simulink model "CRC_8"  (R2018a)
settings: Solver=VariableStepAuto  StartTime=0.0  StopTime=10.0  RelTol=1e-3
values from neighbouring files (symbols this model uses):
  BER = ber(ii)    [CRC_88.m]    (also in RS_77.m)
undefined symbols (not defined in the file or in its folder): CRC
libraries: commcrc2 x2, commrandsrc3 x1, commchan3 x1, dspmathops x1, commsink2 x1
settings Model: Creator=sdf  LastModifiedBy=sdf

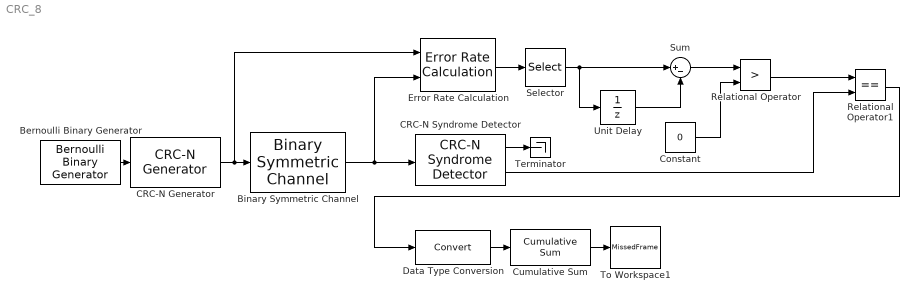
== system CRC_8 ==
  Bernoulli Binary Generator : commrandsrc3/Bernoulli Binary Generator  ProbabilityOfZero=0.5  SeedSource=Parameter  Seed=61  SampleTime=1/640000  SamplesPerFrame=64  OutputDataType=double  SimulateUsing=Interpreted execution
  Binary Symmetric Channel : commchan3/Binary Symmetric Channel  P=BER  s=71  E=off  outDtype=double
      settings: SourceProductName=Communications System Toolbox  SourceProductBaseCode=CM
  CRC-N Generator : commcrc2/CRC-N Generator  crcMethod=CRC-16  iniStates=[0]  numChecksums=1
      settings: SourceProductName=Communications System Toolbox  SourceProductBaseCode=CM
  CRC-N Syndrome Detector : commcrc2/CRC-N Syndrome Detector  crcMethod=CRC-16  iniStates=[0]  numChecksums=1
      settings: SourceProductName=Communications System Toolbox  SourceProductBaseCode=CM
  Constant : Constant  Value=0
  Cumulative Sum : dspmathops/Cumulative Sum  dim=Channels (running sum)  InputProcessing=Columns as channels (frame based)  reset_popup=None  roundingMode=Floor  overflowMode=off  outputDataTypeStr=Inherit: Same as accumulator  outputMin=[]  outputMax=[]  outputLastDataTypeStr=Inherit: Same as accumulator
      settings: SourceProductName=DSP System Toolbox
  Data Type Conversion : DataTypeConversion
  Error Rate Calculation : commsink2/Error Rate Calculation  N=0  st_delay=0  cp_mode=Entire frame  subframe=[]  PMode=Port  WsName=ErrorVec  RsMode2=off  stop=off  numErr=100  maxBits=1e6
  Relational Operator : RelationalOperator  Operator=>  OutDataTypeStr=boolean  RndMeth=Simplest
  Relational Operator1 : RelationalOperator  Operator===  OutDataTypeStr=boolean  RndMeth=Simplest
  Selector : Selector  InputPortWidth=3  IndexOptions=Index vector (dialog)  Indices=[1 3]  OutputSizes=1
  Sum : Sum  Inputs=|+-
  Terminator : Terminator
  To Workspace1 : ToWorkspace  VariableName=MissedFrame  SampleTime=-1
      settings: Save2DSignal=2-D array (concatenate along first dimension)
  Unit Delay : UnitDelay  SampleTime=-1
  wires:
  CRC-N Generator/1 -> Error Rate Calculation/1, Binary Symmetric Channel/1
  Bernoulli Binary Generator/1 -> CRC-N Generator/1
  Binary Symmetric Channel/1 -> Error Rate Calculation/2, CRC-N Syndrome Detector/1
  Error Rate Calculation/1 -> Selector/1
  Selector/1 -> Unit Delay/1, Sum/1
  Unit Delay/1 -> Sum/2
  Sum/1 -> Relational Operator/1
  Constant/1 -> Relational Operator/2
  Relational Operator/1 -> Relational Operator1/1
  CRC-N Syndrome Detector/2 -> Relational Operator1/2
  CRC-N Syndrome Detector/1 -> Terminator/1
  Relational Operator1/1 -> Data Type Conversion/1
  Data Type Conversion/1 -> Cumulative Sum/1
  Cumulative Sum/1 -> To Workspace1/1
